simulink model "HSX_series_cap"  (R2023b)
settings: Solver=VariableStepAuto  StartTime=0.0  StopTime=10.0  RelTol=1e-3
undefined symbols (not defined in the file): DiscIntNeverNeededParam, Kanti, Ki, Kp, LHSX, Ra, RHSX, Ts, Tsamp, Vf
libraries: spsVoltageMeasurementLib x6, spsSeriesRLCBranchLib x6, spsCurrentMeasurementLib x5, spsControlledVoltageSourceLib x2, spsDCMachineLib x2, spsGroundLib x2, spsIdealSwitchLib x2, spsMosfetLib x2, spsDiodeLib x1, spsSawtoothGeneratorLib x1, spsDCVoltageSourceLib x1, sps_lib x1
settings Model: Creator=baik3-ad  LastModifiedBy=baik3-ad

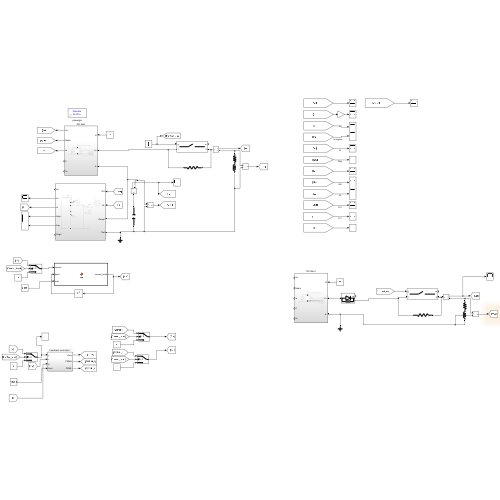
[thumbnail: Simulink's stored preview of the top-level diagram]
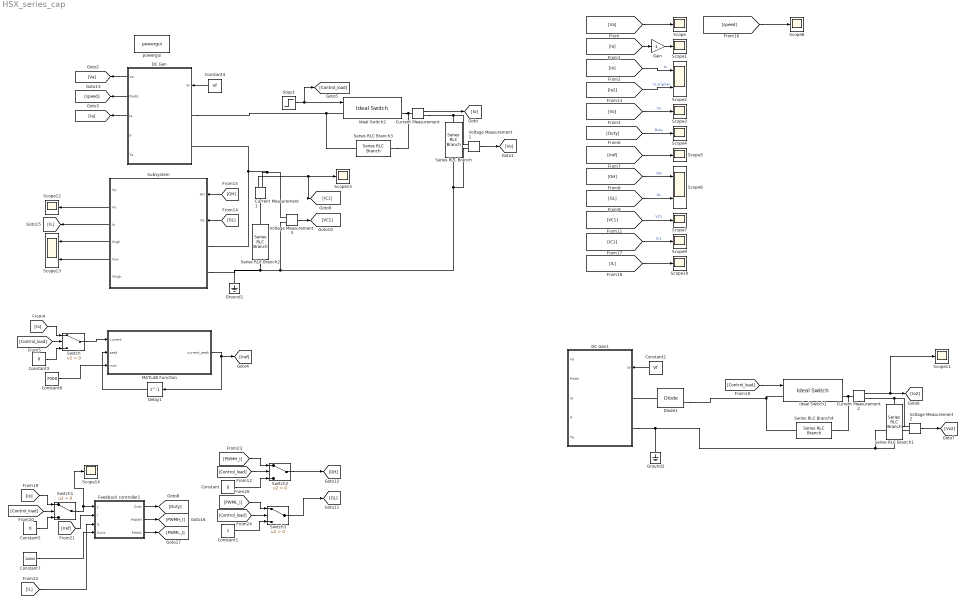
== system HSX_series_cap ==
  Constant : Constant  Value=0
  Constant1 : Constant
  Constant2 : Constant  Value=Vf
  Constant3 : Constant  Value=0
  Constant4 : Constant  Value=Vf
  Constant5 : Constant  Value=0
  Constant6 : Constant  Value=7000
  Constant7 : Constant  Value=10000
  Current Measurement : spsCurrentMeasurementLib/Current Measurement  PhasorSimulation=off  OutputType=Complex  PSBequivalent=0
  Current Measurement1 : spsCurrentMeasurementLib/Current Measurement  PhasorSimulation=off  OutputType=Complex  PSBequivalent=0
  Current Measurement2 : spsCurrentMeasurementLib/Current Measurement  PhasorSimulation=off  OutputType=Complex  PSBequivalent=0
  DC Gen : Subsystem
  DC Gen1 : Subsystem
  Delay1 : Delay  DelayLength=1  InitialCondition=0  SampleTime=Tsamp
  Diode1 : spsDiodeLib/Diode  Ron=0.001  Lon=0  Vf=0.8  IC=0  UseSnubber=0  Rs=500  Cs=250e-9  Measurements=on
  Feedback controller1 : Subsystem
  Gain : Gain  Gain=-1
  Ground1 : spsGroundLib/Ground  LConnTagsString=a
  Ground2 : spsGroundLib/Ground  LConnTagsString=a
  Ideal Switch1 : spsIdealSwitchLib/Ideal Switch  Ron=1e-6  Lon=0  IC=0  Rs=1e8  Cs=0  Measurements=on
  Ideal Switch2 : spsIdealSwitchLib/Ideal Switch  Ron=1e-6  Lon=0  IC=0  Rs=1e8  Cs=0  Measurements=on
  MATLAB Function : MATLAB Function  TreatAsAtomicUnit=on
  Scope{,1,3..5,7..12,14..15} (13 alike) : Scope
  Scope13 : Scope  NumInputPorts=2
  Scope2 : Scope  NumInputPorts=2
  Scope6 : Scope  NumInputPorts=2
  Series RLC Branch : spsSeriesRLCBranchLib/Series RLC Branch  LConnTagsString=__new0  RConnTagsString=__new0  BranchType=RL  Resistance=RHSX  Inductance=LHSX  SetiL0=off  InitialCurrent=0  Capacitance=1e-6  Setx0=off  InitialVoltage=0  Measurements=None
  Series RLC Branch1 : spsSeriesRLCBranchLib/Series RLC Branch  LConnTagsString=__new0  RConnTagsString=__new0  BranchType=RL  Resistance=RHSX  Inductance=LHSX  SetiL0=off  InitialCurrent=0  Capacitance=1e-6  Setx0=off  InitialVoltage=0  Measurements=None
  Series RLC Branch2 : spsSeriesRLCBranchLib/Series RLC Branch  LConnTagsString=__new0  RConnTagsString=__new0  BranchType=C  Resistance=RHSX  Inductance=LHSX  SetiL0=off  InitialCurrent=0  Capacitance=1e-6  Setx0=off  InitialVoltage=0  Measurements=None
  Series RLC Branch3 : spsSeriesRLCBranchLib/Series RLC Branch  LConnTagsString=__new0  RConnTagsString=__new0  BranchType=R  Resistance=1e8  Inductance=0  SetiL0=off  InitialCurrent=0  Capacitance=1e-6  Setx0=off  InitialVoltage=0  Measurements=None
  Series RLC Branch4 : spsSeriesRLCBranchLib/Series RLC Branch  LConnTagsString=__new0  RConnTagsString=__new0  BranchType=R  Resistance=1e8  Inductance=0  SetiL0=off  InitialCurrent=0  Capacitance=1e-6  Setx0=off  InitialVoltage=0  Measurements=None
  Step3 : Step  Time=4  SampleTime=0  VectorParams1D=off  ZeroCross=off
  Subsystem : Subsystem
  Switch{,1..3} (4 alike) : Switch  Criteria=u2 > Threshold  SaturateOnIntegerOverflow=off  InputSameDT=off
  Voltage Measurement1 : spsVoltageMeasurementLib/Voltage Measurement  PhasorSimulation=off  OutputType=Complex  PSBequivalent=0
  Voltage Measurement2 : spsVoltageMeasurementLib/Voltage Measurement  PhasorSimulation=off  OutputType=Complex  PSBequivalent=0
  Voltage Measurement3 : spsVoltageMeasurementLib/Voltage Measurement  PhasorSimulation=off  OutputType=Complex  PSBequivalent=0
  powergui : sps_lib/powergui  Priority=1  SimulationMode=Discrete  SampleTime=Tsamp  frequency=60  Iterations=50  frequencyindice=0  Pbase=100e6  ErrMax=1e-4  UnitsV=kV  UnitsW=MW  buscounter=0  FunctionMessages=off  echomessages=off  EnableUseOfTLC=off  CurrentSourceSwitches=off  DisableSnubberDevices=off  DisableRonSwitches=off  DisableVfSwitches=off  DisplayEquations=off  AutomaticDiscreteSolvers=off  SolverType=Tustin/Backward Euler (TBE)  Interpol=off  ExternalGateDelay=off  methode=off  Ts=100  x0status=blocks  SPID=on  SwTol=0  HookPort=off  NonlinearTolerance=1e-4  nMaxIteration=100  ContinueOnMaxIteration=off  RestoreLinks=warning  ResistiveCurrentMeasurement=off  Frange=[0:2:500]  Ylog=off  Xlog=on  ShowGrid=off  save=off  variable=ZData  structure=0  ZoomFFT=off  StartTime=0.0  cycles=1  DisplayStyle=1  fundamental=60  FreqAxis=off  MaxFrequency=1000  frequencyindicesteady=1  RmsSteady=1  display=off
  wires:
  Constant4/1 -> DC Gen/1(Vf)
  Step3/1 -> [Control_load], Ideal Switch2/1
  Current Measurement/1 -> [Io]
  Voltage Measurement1/1 -> [Vo]
  DC Gen/1(Va) -> [Va]
  DC Gen/3(Ia) -> [Ia]
  [Va] -> Scope/1
  [Io] -> Scope2/1  "Io"
  [Vo] -> Scope3/1  "Vo"
  [Ia] -> Gain/1
  Gain/1 -> Scope1/1
  MATLAB Function/1(current_peak) -> [Iref], Delay1/1
  Delay1/1 -> MATLAB Function/2(peak)
  [Iref] -> Scope5/1
  [GH] -> Scope6/1  "GH"
  [GL] -> Scope6/2  "GL"
  Voltage Measurement3/1 -> [VC1]
  [VC1] -> Scope7/1  "VC1"
  Switch2/1 -> [GH]
  Switch3/1 -> [GL]
  [GL] -> Subsystem/2(GL)
  [GH] -> Subsystem/1(GH)
  DC Gen/2(Rad/s) -> [speed]
  [speed] -> Scope8/1
  [IC1] -> Scope9/1  "IC1"
  Subsystem/3(Io) -> [IL]
  [IL] -> Scope10/1
  Subsystem/2(Vo) -> Scope12/1
  Subsystem/4(Ihigh) -> Scope13/1
  Subsystem/5(Ilow) -> Scope13/2
  [Control_load] -> Switch/2
  Switch/1 -> MATLAB Function/1(current)
  [Io] -> Switch/1
  Constant3/1 -> Switch/3
  [Control_load] -> Switch1/2
  Constant5/1 -> Switch1/3
  [Io] -> Switch1/1
  Switch1/1 -> Scope14/1, Feedback controller1/1(y)
  [Iref] -> Feedback controller1/2(r)
  Feedback controller1/1(Duty) -> [Duty]
  [Control_load] -> Switch2/2
  [PWMH_I] -> Switch2/1
  Constant/1 -> Switch2/3
  [PWML_I] -> Switch3/1
  Constant1/1 -> Switch3/3
  [Control_load] -> Switch3/2
  Current Measurement2/1 -> Scope11/1, [Io2]
  Constant2/1 -> DC Gen1/1(Vf)
  Voltage Measurement2/1 -> [Vo2]
  [Control_load] -> Ideal Switch1/1
  [Io2] -> Scope2/2  "Io original"
  [Duty] -> Scope4/1  "Duty"
  Constant6/1 -> MATLAB Function/3(max)
  [IL] -> Feedback controller1/3(IL)
  Constant7/1 -> Feedback controller1/4(Ilimit)
  Feedback controller1/3(PWML) -> [PWML_I]
  Feedback controller1/2(PWMH) -> [PWMH_I]
  Current Measurement1/1 -> [IC1], Scope15/1
  connections:
  Subsystem/LConn2 -- Ground1/LConn1 -- Series RLC Branch2/RConn1 -- Voltage Measurement3/LConn2 -- Series RLC Branch/RConn1 -- Voltage Measurement1/LConn2
  Voltage Measurement1/LConn1 -- Current Measurement/RConn1 -- Series RLC Branch/LConn1
  Current Measurement/LConn1 -- Series RLC Branch3/LConn1 -- Ideal Switch2/RConn1
  Ideal Switch1/LConn1 -- Diode1/RConn1 -- Series RLC Branch4/RConn1
  Ideal Switch1/RConn1 -- Current Measurement2/LConn1 -- Series RLC Branch4/LConn1
  Series RLC Branch1/LConn1 -- Voltage Measurement2/LConn1 -- Current Measurement2/RConn1
  Diode1/LConn1 -- DC Gen1/LConn1
  DC Gen1/LConn2 -- Series RLC Branch1/RConn1 -- Voltage Measurement2/LConn2 -- Ground2/LConn1
  Ideal Switch2/LConn1 -- DC Gen/LConn1 -- Series RLC Branch3/RConn1
  Voltage Measurement3/LConn1 -- Current Measurement1/RConn1 -- Subsystem/LConn1 -- DC Gen/LConn2
  Current Measurement1/LConn1 -- Series RLC Branch2/LConn1

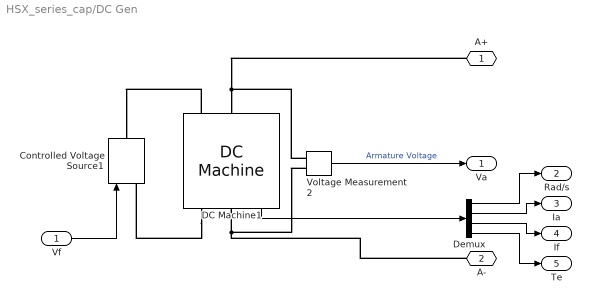
== system HSX_series_cap/DC Gen ==
  Vf : Inport
  Controlled Voltage Source1 : spsControlledVoltageSourceLib/Controlled Voltage Source  Initialize=on  Source_Type=DC  Amplitude=0  Phase=0  Frequency=0  Measurements=Voltage
  DC Machine1 : spsDCMachineLib/DC Machine  PresetModel=No  MechanicalLoad=Torque TL  FieldType=Wound  ShowDetailedParameters=on  MeasurementBus=off  RLa="[Ra  0.002]"  RLf=[0.0054 0.0125]  Laf=Laf  MachineConstant=Torque constant (N.m/A)  Ke=1.8  Kt=1.8  J=137  Bm=0  Tf=0  w0=w_initial  Ifinit=0  TsPowergui=0  TsBlock=-1
  Demux : Demux
  Voltage Measurement2 : spsVoltageMeasurementLib/Voltage Measurement  PhasorSimulation=off  OutputType=Complex  PSBequivalent=0
  A+ : PMIOPort  Side=Left
  A- : PMIOPort  Port=2  Side=Left
  Va : Outport
  Rad/s : Outport  Port=2
  Ia : Outport  Port=3
  If : Outport  Port=4
  Te : Outport  Port=5
  wires:
  DC Machine1/1 -> Demux/1
  Vf/1 -> Controlled Voltage Source1/1
  Voltage Measurement2/1 -> Va/1  "Armature Voltage"
  Demux/1 -> Rad/s/1
  Demux/4 -> Te/1
  Demux/3 -> If/1
  Demux/2 -> Ia/1
  connections:
  Voltage Measurement2/LConn1 -- A+/RConn1 -- DC Machine1/LConn1
  A-/RConn1 -- Voltage Measurement2/LConn2 -- DC Machine1/RConn1
  DC Machine1/LConn2 -- Controlled Voltage Source1/RConn1
  DC Machine1/RConn2 -- Controlled Voltage Source1/LConn1

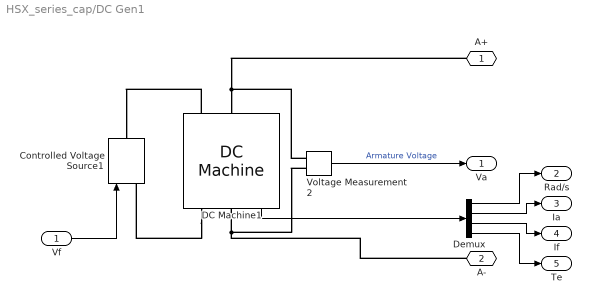
== system HSX_series_cap/DC Gen1 ==
  Vf : Inport
  Controlled Voltage Source1 : spsControlledVoltageSourceLib/Controlled Voltage Source  Initialize=on  Source_Type=DC  Amplitude=0  Phase=0  Frequency=0  Measurements=Voltage
  DC Machine1 : spsDCMachineLib/DC Machine  PresetModel=No  MechanicalLoad=Torque TL  FieldType=Wound  ShowDetailedParameters=on  MeasurementBus=off  RLa="[Ra  0.002]"  RLf=[0.0054 0.0125]  Laf=Laf  MachineConstant=Torque constant (N.m/A)  Ke=1.8  Kt=1.8  J=137  Bm=0  Tf=0  w0=w_initial  Ifinit=0  TsPowergui=0  TsBlock=-1
  Demux : Demux
  Voltage Measurement2 : spsVoltageMeasurementLib/Voltage Measurement  PhasorSimulation=off  OutputType=Complex  PSBequivalent=0
  A+ : PMIOPort  Side=Left
  A- : PMIOPort  Port=2  Side=Left
  Va : Outport
  Rad/s : Outport  Port=2
  Ia : Outport  Port=3
  If : Outport  Port=4
  Te : Outport  Port=5
  wires:
  DC Machine1/1 -> Demux/1
  Vf/1 -> Controlled Voltage Source1/1
  Voltage Measurement2/1 -> Va/1  "Armature Voltage"
  Demux/1 -> Rad/s/1
  Demux/4 -> Te/1
  Demux/3 -> If/1
  Demux/2 -> Ia/1
  connections:
  Voltage Measurement2/LConn1 -- A+/RConn1 -- DC Machine1/LConn1
  A-/RConn1 -- Voltage Measurement2/LConn2 -- DC Machine1/RConn1
  DC Machine1/LConn2 -- Controlled Voltage Source1/RConn1
  DC Machine1/RConn2 -- Controlled Voltage Source1/LConn1

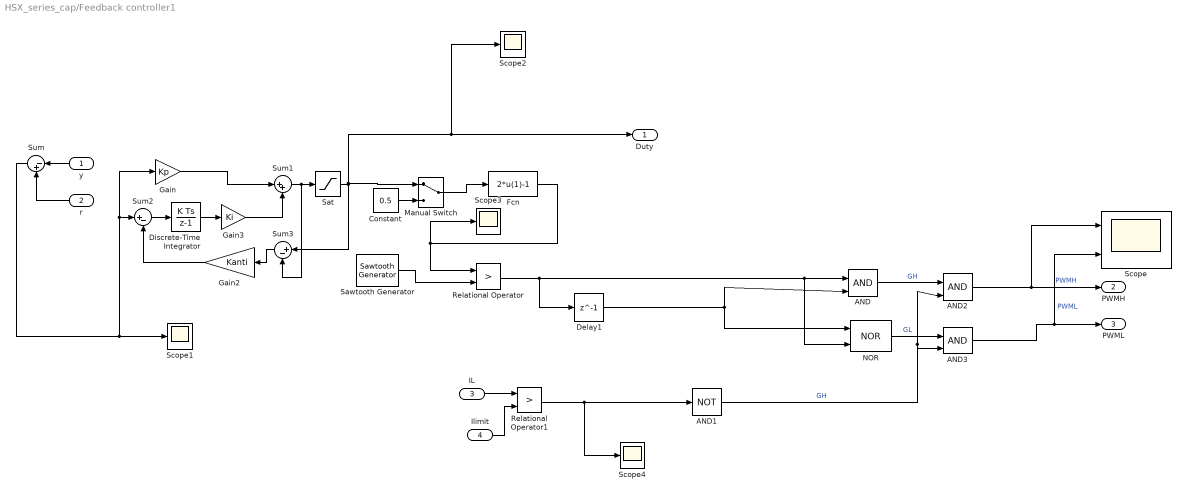
== system HSX_series_cap/Feedback controller1 ==
  y : Inport
  r : Inport  Port=2
  IL : Inport  Port=3
  Ilimit : Inport  Port=4
  AND : Logic  IconShape=distinctive  AllPortsSameDT=off  OutDataTypeStr=boolean
  AND1 : Logic  Operator=NOT  IconShape=distinctive  AllPortsSameDT=off  OutDataTypeStr=boolean
  AND2 : Logic  IconShape=distinctive  AllPortsSameDT=off  OutDataTypeStr=boolean
  AND3 : Logic  IconShape=distinctive  AllPortsSameDT=off  OutDataTypeStr=boolean
  Constant : Constant  Value=0.5
  Delay1 : Delay  DelayLength=1  InitialCondition=0  SampleTime=Tsamp
  Discrete-Time Integrator : DiscreteIntegrator  SampleTime=Tsamp  ICPrevOutput=DiscIntNeverNeededParam  ICPrevScaledInput=DiscIntNeverNeededParam
  Fcn : Fcn  Expr=2*u(1)-1
  Gain : Gain  Gain=Kp
  Gain2 : Gain  Gain=Kanti
  Gain3 : Gain  Gain=Ki
  Manual Switch : ManualSwitch
  NOR : Logic  Operator=NOR  IconShape=distinctive  AllPortsSameDT=off
  Relational Operator : RelationalOperator  Operator=>  OutDataTypeStr=boolean  RndMeth=Simplest  InputSameDT=off
  Relational Operator1 : RelationalOperator  Operator=>  OutDataTypeStr=boolean  RndMeth=Simplest  InputSameDT=off
  Sat : Saturate  UpperLimit=1  LowerLimit=0
  Sawtooth Generator : spsSawtoothGeneratorLib/Sawtooth Generator  Freq=1/Ts  Phase=0  Ts=Tsamp
  Scope : Scope  NumInputPorts=2
  Scope{1..4} (4 alike) : Scope
  Sum : Sum  Inputs=|-+  InputSameDT=on  SaturateOnIntegerOverflow=on  OutDataTypeStr=Inherit: Same as first input
  Sum1 : Sum  Inputs=|++
  Sum2 : Sum  Inputs=|+-
  Sum3 : Sum  Inputs=|+-
  Duty : Outport  VectorParamsAs1DForOutWhenUnconnected=off
  PWMH : Outport  Port=2  VectorParamsAs1DForOutWhenUnconnected=off
  PWML : Outport  Port=3  VectorParamsAs1DForOutWhenUnconnected=off
  wires:
  Sum/1 -> Scope1/1, Gain/1, Sum2/1
  y/1 -> Sum/1
  r/1 -> Sum/2
  Sat/1 -> Sum3/1, Manual Switch/1, Scope2/1, Duty/1
  Sum1/1 -> Sum3/2, Sat/1
  Gain/1 -> Sum1/1
  Sum2/1 -> Discrete-Time Integrator/1
  Sum3/1 -> Gain2/1
  Gain2/1 -> Sum2/2
  Sawtooth Generator/1 -> Relational Operator/2
  Relational Operator/1 -> Delay1/1, NOR/2, AND/1
  Delay1/1 -> NOR/1, AND/2
  Fcn/1 -> Scope3/1, Relational Operator/1
  Discrete-Time Integrator/1 -> Gain3/1
  Gain3/1 -> Sum1/2
  IL/1 -> Relational Operator1/1
  Ilimit/1 -> Relational Operator1/2
  AND/1 -> AND2/1  "GH"
  AND2/1 -> Scope/1, PWMH/1  "PWMH"
  AND3/1 -> PWML/1, Scope/2  "PWML"
  NOR/1 -> AND3/1  "GL"
  Relational Operator1/1 -> Scope4/1, AND1/1
  AND1/1 -> AND3/2, AND2/2  "GH"
  Manual Switch/1 -> Fcn/1
  Constant/1 -> Manual Switch/2

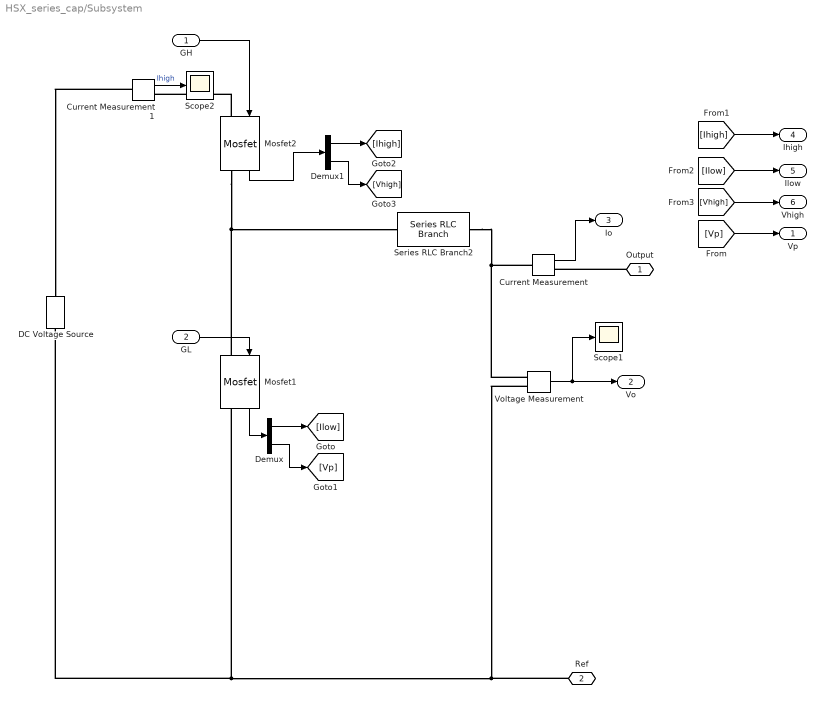
== system HSX_series_cap/Subsystem ==
  GH : Inport
  GL : Inport  Port=2
  Current Measurement : spsCurrentMeasurementLib/Current Measurement  PhasorSimulation=off  OutputType=Complex  PSBequivalent=0
  Current Measurement1 : spsCurrentMeasurementLib/Current Measurement  PhasorSimulation=off  OutputType=Complex  PSBequivalent=0
  DC Voltage Source : spsDCVoltageSourceLib/DC Voltage Source  Amplitude=100  Measurements=None
  Demux : Demux  Outputs=2
  Demux1 : Demux  Outputs=2
  Mosfet1 : spsMosfetLib/Mosfet  Ron=0.0001  Lon=0  Rd=0.0001  Vfd=0  IC=0  Rs=1e5  Cs=inf  Measurements=on
  Mosfet2 : spsMosfetLib/Mosfet  Ron=0.0001  Lon=0  Rd=0.0001  Vfd=0  IC=0  Rs=1e5  Cs=inf  Measurements=on
  Scope1 : Scope
  Scope2 : Scope
  Series RLC Branch2 : spsSeriesRLCBranchLib/Series RLC Branch  LConnTagsString=__new0  RConnTagsString=__new0  BranchType=L  Resistance=0.09  Inductance=1e-3  SetiL0=on  InitialCurrent=0  Capacitance=1e-1  Setx0=off  InitialVoltage=0  Measurements=None
  Voltage Measurement : spsVoltageMeasurementLib/Voltage Measurement  PhasorSimulation=off  OutputType=Complex  PSBequivalent=0
  Output : PMIOPort  Side=Left
  Ref : PMIOPort  Port=2  Side=Left
  Vp : Outport
  Vo : Outport  Port=2
  Io : Outport  Port=3
  Ihigh : Outport  Port=4
  Ilow : Outport  Port=5
  Vhigh : Outport  Port=6
  wires:
  Voltage Measurement/1 -> Vo/1, Scope1/1
  GL/1 -> Mosfet1/1
  Current Measurement/1 -> Io/1
  Mosfet1/1 -> Demux/1
  Demux/1 -> [Ilow]
  Demux/2 -> [Vp]
  [Vp] -> Vp/1
  GH/1 -> Mosfet2/1
  Demux1/2 -> [Vhigh]
  Mosfet2/1 -> Demux1/1
  Demux1/1 -> [Ihigh]
  [Ihigh] -> Ihigh/1
  [Ilow] -> Ilow/1
  [Vhigh] -> Vhigh/1
  Current Measurement1/1 -> Scope2/1  "Ihigh"
  connections:
  Series RLC Branch2/RConn1 -- Current Measurement/LConn1 -- Voltage Measurement/LConn1
  Mosfet1/LConn1 -- Mosfet2/RConn1 -- Series RLC Branch2/LConn1
  Voltage Measurement/LConn2 -- Ref/RConn1 -- DC Voltage Source/LConn1 -- Mosfet1/RConn1
  Output/RConn1 -- Current Measurement/RConn1
  Current Measurement1/LConn1 -- DC Voltage Source/RConn1
  Mosfet2/LConn1 -- Current Measurement1/RConn1

== matlab function HSX_series_cap/MATLAB Function ==
  data: current input; current_peak output; peak input; max input
function current_peak = fcn(current, peak,max)
    if current>peak
        current_peak = current;
    else
        current_peak = peak;
    end

    if (max ~= 0)&&(peak>=max)
        current_peak = max;
     
    end
